simulink library "FUSA_EM_EMRR"  (R2023b)
settings: Solver=VariableStepAuto  StartTime=0.0  StopTime=10.0  RelTol=1e-3
undefined symbols (not defined in the file): FUSA_EM_EMRR_p1_TempMotDertCoefReRi_na, FUSA_EM_EMRR_px_TempMotReRiLkp_degC
libraries: simulink x1
settings Model: Creator=blatak  LastModifiedBy=blatak

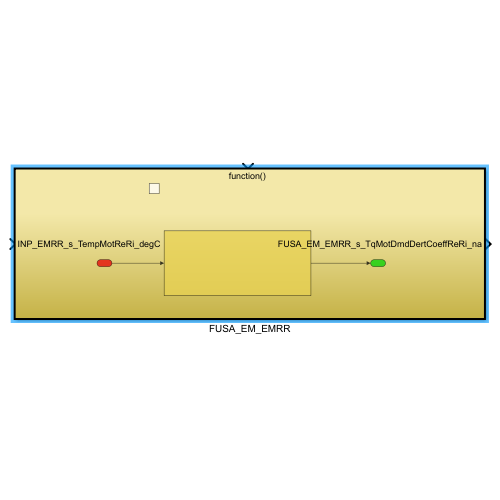
[thumbnail: Simulink's stored preview of the top-level diagram]
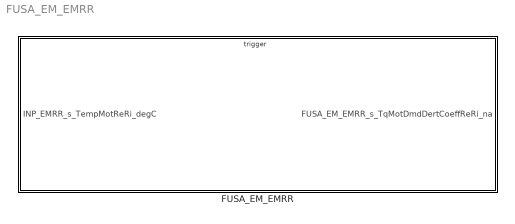
== system FUSA_EM_EMRR ==
  FUSA_EM_EMRR : Subsystem  TreatAsAtomicUnit=on

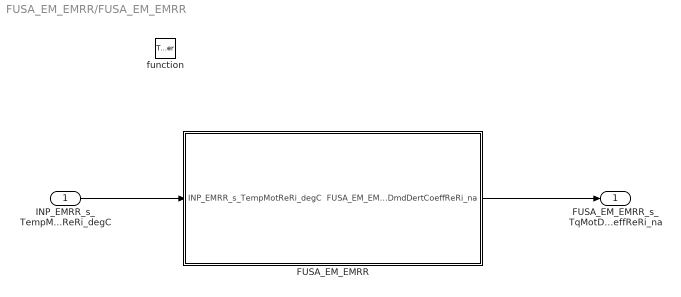
== system FUSA_EM_EMRR/FUSA_EM_EMRR ==
  INP_EMRR_s_TempMotReRi_degC : Inport
  function : TriggerPort  TriggerType=function-call  VariantControl=(inherit)
  FUSA_EM_EMRR : Subsystem
  FUSA_EM_EMRR_s_TqMotDmdDertCoeffReRi_na : Outport  Description=Derate torque coefficient front
  wires:
  INP_EMRR_s_TempMotReRi_degC/1 -> FUSA_EM_EMRR/1(INP_EMRR_s_TempMotReRi_degC)
  FUSA_EM_EMRR/1(FUSA_EM_EMRR_s_TqMotDmdDertCoeffReRi_na) -> FUSA_EM_EMRR_s_TqMotDmdDertCoeffReRi_na/1

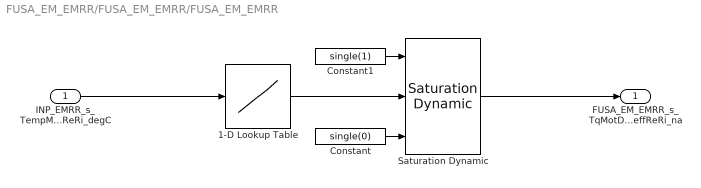
== system FUSA_EM_EMRR/FUSA_EM_EMRR/FUSA_EM_EMRR ==
  INP_EMRR_s_TempMotReRi_degC : Inport
  1-D Lookup Table : Lookup_n-D  NumberOfTableDimensions=1  BreakpointsForDimension1=FUSA_EM_EMRR_px_TempMotReRiLkp_degC  Table=FUSA_EM_EMRR_p1_TempMotDertCoefReRi_na  InternalRulePriority=Speed  RndMeth=Simplest
  Constant : Constant  Value=single(0)
  Constant1 : Constant  Value=single(1)
  Saturation Dynamic : simulink/Discontinuities/Saturation Dynamic  OutMin=[]  OutMax=[]  OutDataTypeStr=Inherit: Same as second input  OutDataType=fixdt(1, 16)  OutScaling=2^-10  DoSatur=off
  FUSA_EM_EMRR_s_TqMotDmdDertCoeffReRi_na : Outport  Description=Derate torque coefficient front
  wires:
  Saturation Dynamic/1 -> FUSA_EM_EMRR_s_TqMotDmdDertCoeffReRi_na/1
  Constant1/1 -> Saturation Dynamic/1
  1-D Lookup Table/1 -> Saturation Dynamic/2
  INP_EMRR_s_TempMotReRi_degC/1 -> 1-D Lookup Table/1
  Constant/1 -> Saturation Dynamic/3
